simulink model "observer"  (R2021b)
settings: Solver=VariableStepAuto  StartTime=0.0  StopTime=10.0  RelTol=1e-3
settings Model: Creator=mfuser  LastModifiedBy=mfuser

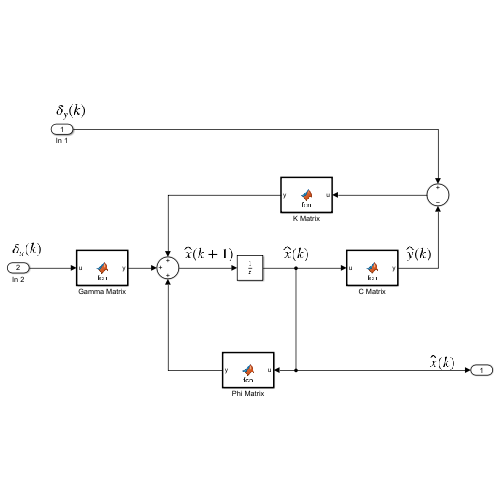
[thumbnail: Simulink's stored preview of the top-level diagram]
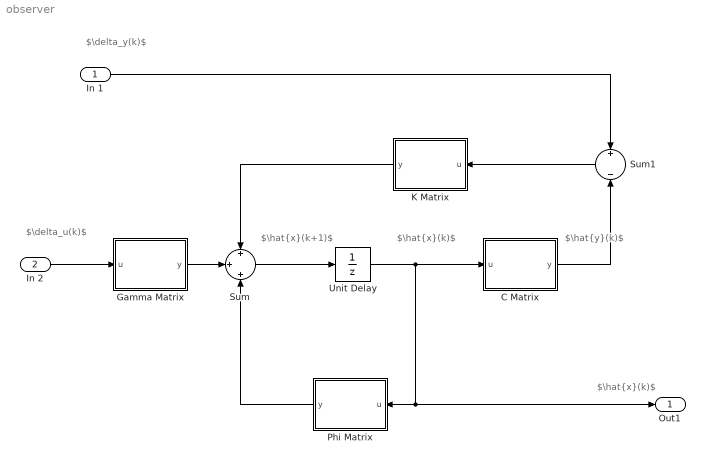
== system observer ==
  note: $\delta_y(k)$
  note: $\delta_u(k)$
  note: $\hat{y}(k)$
  note: $\hat{x}(k)$
  note: $\hat{x}(k+1)$
  note: $\hat{x}(k)$
  In 1 : Inport
  In 2 : Inport  Port=2
  C Matrix : MATLAB Function  TreatAsAtomicUnit=on
  Gamma Matrix : MATLAB Function  TreatAsAtomicUnit=on
  K Matrix : MATLAB Function  TreatAsAtomicUnit=on
  Phi Matrix : MATLAB Function  TreatAsAtomicUnit=on
  Sum : Sum  Inputs=+|+|+
  Sum1 : Sum  Inputs=+||-
  Unit Delay : UnitDelay  SampleTime=-1  HasFrameUpgradeWarning=on
  Out1 : Outport
  wires:
  Phi Matrix/1(y) -> Sum/3
  Gamma Matrix/1(y) -> Sum/2
  Sum/1 -> Unit Delay/1
  Unit Delay/1 -> Out1/1, Phi Matrix/1(u), C Matrix/1(u)
  C Matrix/1(y) -> Sum1/2
  Sum1/1 -> K Matrix/1(u)
  K Matrix/1(y) -> Sum/1
  In 1/1 -> Sum1/1
  In 2/1 -> Gamma Matrix/1(u)

== matlab function observer/C Matrix ==
  data: u input; y output; C_discr parameter
function y = fcn(u, C_discr)

y = C_discr*u;

== matlab function observer/Gamma Matrix ==
  data: u input; y output; B_discr parameter
function y = fcn(u, B_discr)

y = B_discr*u;

== matlab function observer/K Matrix ==
  data: u input; y output; K_matrix parameter
function y = fcn(u, K_matrix)

y = K_matrix*u;

== matlab function observer/Phi Matrix ==
  data: u input; y output; A_discr parameter
function y = fcn(u, A_discr)

y = A_discr*u;
